simulink model "Race_Control"  (R2015a)
settings: Solver=ode3  SolverMode=SingleTasking  StartTime=0.0  StopTime=inf  FixedStep=0.001  MaxStep=0.004  RelTol=1e-3
undefined symbols (not defined in the file): obstacles, obstacles_AABB, quadrotor_AABB, waypoints
libraries: dspsigops x2
settings Model: CovSFcnEnable=off  Creator=ADAM  LastModifiedBy=denise
settings SolverCC: ExtrapolationOrder=1
settings DataIOCC: LimitDataPoints=off  MaxDataPoints=1  SaveFormat=Structure  SignalLoggingSaveFormat=ModelDataLogs  SaveOutput=off  SignalLogging=off  DSMLogging=off  SaveTime=off  OutputSaveName=model_out  SignalLoggingName=model_out
settings OptimizationCC: ExpressionDepthLimit=2147483647  SimCompilerOptimization=on
settings DebuggingCC: SolverPrmCheckMsg=warning  InheritedTsInSrcMsg=none  MultiTaskDSMMsg=warning  MultiTaskCondExecSysMsg=none  UnconnectedInputMsg=none  UnconnectedOutputMsg=none  UnconnectedLineMsg=none  StateNameClashWarn=warning
settings HardwareCC: ProdIntDivRoundTo=Zero  ProdEndianess=LittleEndian  ProdHWDeviceType=Generic->32-bit x86 compatible
settings CodeAppCC: MaxIdLength=95

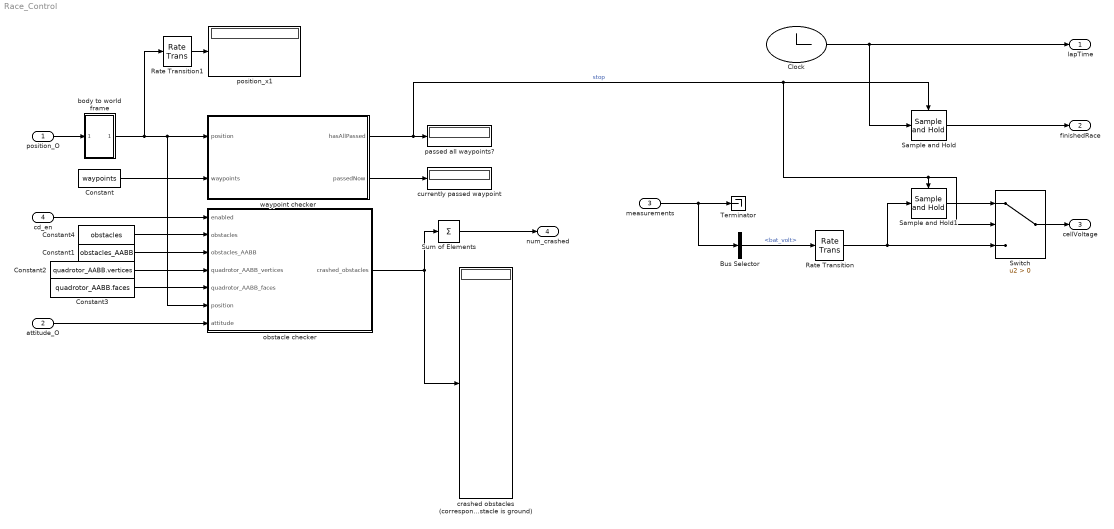
== system Race_Control ==
  position_O : Inport  OutDataTypeStr=double  PortDimensions=3  SampleTime=[0 0]  Interpolate=off
  attitude_O : Inport  Port=2  OutDataTypeStr=double  PortDimensions=4  SampleTime=[0 0]  Interpolate=off
  measurements : Inport  Port=3  OutDataTypeStr=Bus: Sensor_Bus  SampleTime=0.004  Interpolate=off
  cd_en : Inport  Port=4  OutDataTypeStr=boolean  PortDimensions=1  SampleTime=[0 0]  Interpolate=off
  Bus Selector : BusSelector  OutputSignals=bat_volt
  Clock : Clock
      settings: Decimation=4
  Constant : Constant  Value=waypoints  VectorParams1D=off
  Constant1 : Constant  Value=obstacles_AABB  VectorParams1D=off
  Constant2 : Constant  Value=quadrotor_AABB.vertices  VectorParams1D=off
  Constant3 : Constant  Value=quadrotor_AABB.faces  VectorParams1D=off
  Constant4 : Constant  Value=obstacles  VectorParams1D=off
  Rate Transition : RateTransition
  Rate Transition1 : RateTransition
  Sample and Hold : dspsigops/Sample and Hold  trig=Rising edge  initCond=0  latchinput=off
  Sample and Hold1 : dspsigops/Sample and Hold  trig=Rising edge  initCond=0  latchinput=off
  Sum of Elements : Sum  Inputs=+
  Switch : Switch  Criteria=u2 > Threshold
  Terminator : Terminator
  body to world frame : Subsystem
  "crashed obstacles (corresponds to the index of the obstacles defined in the workspace, last obstacle is ground)" : Display
  currently passed waypoint : Display
  obstacle checker : MATLAB Function  TreatAsAtomicUnit=on
  passed all waypoints? : Display
  position_x1 : Display
      settings: Format=decimal (Stored Integer)
  waypoint checker : MATLAB Function  TreatAsAtomicUnit=on
  lapTime : Outport  PortDimensions=1
  finishedRace : Outport  Port=2  PortDimensions=1
  cellVoltage : Outport  Port=3  PortDimensions=1
  num_crashed : Outport  Port=4  PortDimensions=1
  wires:
  waypoint checker/1(hasAllPassed) -> Sample and Hold1/Trigger, Switch/2, Sample and Hold/Trigger, passed all waypoints?/1  "stop"
  Constant/1 -> waypoint checker/2(waypoints)
  attitude_O/1 -> obstacle checker/7(attitude)
  waypoint checker/2(passedNow) -> currently passed waypoint/1
  Constant1/1 -> obstacle checker/3(obstacles_AABB)
  Constant2/1 -> obstacle checker/4(quadrotor_AABB_vertices)
  obstacle checker/1(crashed_obstacles) -> "crashed obstacles (corresponds to the index of the obstacles defined in the workspace, last obstacle is ground)"/1, Sum of Elements/1
  Constant3/1 -> obstacle checker/5(quadrotor_AABB_faces)
  measurements/1 -> Bus Selector/1, Terminator/1
  Bus Selector/1 -> Rate Transition/1  "<bat_volt>"
  Clock/1 -> Sample and Hold/1, lapTime/1
  Sample and Hold/1 -> finishedRace/1
  Sample and Hold1/1 -> Switch/1
  Rate Transition/1 -> Sample and Hold1/1, Switch/3
  Rate Transition1/1 -> position_x1/1
  body to world frame/1(world) -> Rate Transition1/1, obstacle checker/6(position), waypoint checker/1(position)
  position_O/1 -> body to world frame/1(NED)
  cd_en/1 -> obstacle checker/1(enabled)
  Constant4/1 -> obstacle checker/2(obstacles)
  Sum of Elements/1 -> num_crashed/1
  Switch/1 -> cellVoltage/1

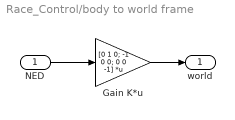
== system Race_Control/body to world frame ==
  NED : Inport
  Gain K*u : Gain  Gain=[0 1 0; -1 0 0; 0 0 -1]  Multiplication=Matrix(K*u)
  world : Outport
  wires:
  NED/1 -> Gain K*u/1
  Gain K*u/1 -> world/1

== matlab function Race_Control/obstacle checker ==
  data: enabled input; obstacles input; obstacles_AABB input; quadrotor_AABB_vertices input; quadrotor_AABB_faces input; position input; attitude input; crashed_obstacles output
 function crashed_obstacles = obstacleChecker( enabled, obstacles, obstacles_AABB, quadrotor_AABB_vertices, quadrotor_AABB_faces, position, attitude )
%OBSTACLECHECKER Returns a vector indicated which obstacles have been collided with. 
%   
%   obstacles_AABB The axis-aligned bounding boxes of the obstacles.
%   quadrotor_AABB The axis-aligned bounding box of the quadrotor. This
%   bounding box will be transformed w.r.t. given position and attitude.
%   position The position of the quadrotor, described by a 3-dim vector
%   [x;y;z].
%   attitude The rotation of the quadrotor, described by a 3-dim array or
%   vector [roll pitch yaw] or a quaternion, a 4-dim array [q0 q1 q2 q3].
%
%   Returns:
%   crashed_obstacles Boolean vector that indicates which obstacles have
%   been crashed.
%   Note: last obstacle in that vector is the ground, assumed at hight
%   zero.

qr_AABB.vertices = quadrotor_AABB_vertices;
qr_AABB.faces = quadrotor_AABB_faces;
crashed_obstacles = zeros(length(obstacles)+1, 1); % needed to define the output size of this function
if enabled
    crashed_obstacles = hasCrashedObstacle(obstacles, obstacles_AABB, qr_AABB, position, attitude);
end
end

== matlab function Race_Control/waypoint checker ==
  data: position input; hasAllPassed output; waypoints input; passedNow output
function [hasAllPassed, passedNow] = waypointChecker(position, waypoints)
%HASPASSEDWAYPOINTS Returns true if all waypoints have been passed, otherwise false.
%
%   position The position of the quadrotor, described by a 3-dim vector
%   [x;y;z].
%   waypoints The position of waypoints as a matrix. Each row holds the
%   position of a waypoint as [x y z].
%
%   hasAllPassed A boolean indicating if all waypoints have been passed.
%   passedNow The index of the waypoint in matrix waypoints that is catched
%   at this moment.
%
%   If a waypoint is passed, i.e., the distance between quadrotor and the
%   center of the waypoint is smaller than the waypoint's radius, an
%   appropriate waypoint flag is set. When all flags are set this function
%   returns true.
%
%   Note the radius is hardcoded here. So check the radius of a waypoint in
%   initWorld.m.

[hasAllPassed, passedNow] = hasPassedWaypoints(position, waypoints);

end
